simulink model "forward_acceleration_model"  (R2020a)
settings: Solver=VariableStepAuto  StartTime=0.0  StopTime=10.0  RelTol=1e-3
settings Model: Creator=Lord  LastModifiedBy=Lord

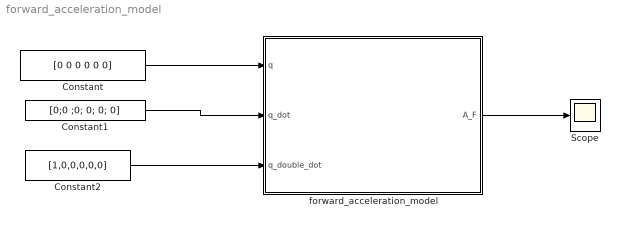
== system forward_acceleration_model ==
  Constant : Constant  Value=[0 0 0 0 0 0]
  Constant1 : Constant  Value=[0;0 ;0; 0; 0; 0]
  Constant2 : Constant  Value=[1,0,0,0,0,0]
  Scope : Scope
  forward_acceleration_model : MATLAB Function  TreatAsAtomicUnit=on
  wires:
  Constant/1 -> forward_acceleration_model/1(q)
  Constant1/1 -> forward_acceleration_model/2(q_dot)
  Constant2/1 -> forward_acceleration_model/3(q_double_dot)
  forward_acceleration_model/1(A_F) -> Scope/1

== matlab function forward_acceleration_model/forward_acceleration_model ==
  data: q input; A_F output; q_dot input; q_double_dot input
function  A_F = forward_acceleration_model(q,q_dot,q_double_dot)
  
A_F=zeros(6,1);
J = jacobian_matrix_num(q);
J_dot = jacobian_derivative_num(q,q_dot);

A_F = (J_dot*q_dot)+(J*transpose(transpose(q_double_dot)));

end
